simulink model "HDLOFDMMod"  (R2024a)
settings: Solver=FixedStepDiscrete  StartTime=0.0  StopTime=stopTime  RelTol=1e-3
undefined symbols (not defined in the file): CONST, dataSymbols
libraries: dspsrcs4 x2, HDL_ieee_8021513 x2, hdlsllib x1, whdlutilities x1
settings Model: DataTypeOverride=Off  Creator=cotti  LastModifiedBy=cotti
settings OptimizationCC: BlockReduction=off  ConditionallyExecuteInputs=off  DefaultParameterBehavior=Inlined  InheritOutputTypeSmallerThanSingle=on
settings DebuggingCC: ArtificialAlgebraicLoopMsg=error  SingleTaskRateTransMsg=error
settings HardwareCC: ProdBitPerPointer=32  ProdBitPerSizeT=32  ProdBitPerPtrDiffT=32  ProdLargestAtomicFloat=None  ProdIntDivRoundTo=Undefined  ProdEndianess=Unspecified  ProdWordSize=32  ProdHWDeviceType=ASIC/FPGA->ASIC/FPGA  TargetBitPerLong=64  TargetBitPerPointer=64  TargetBitPerSizeT=64  TargetBitPerPtrDiffT=64  TargetLongLongMode=on  TargetIntDivRoundTo=Zero  TargetEndianess=LittleEndian  TargetWordSize=64  TargetHWDeviceType=Custom Processor->MATLAB Host Computer  ProdEqTarget=off

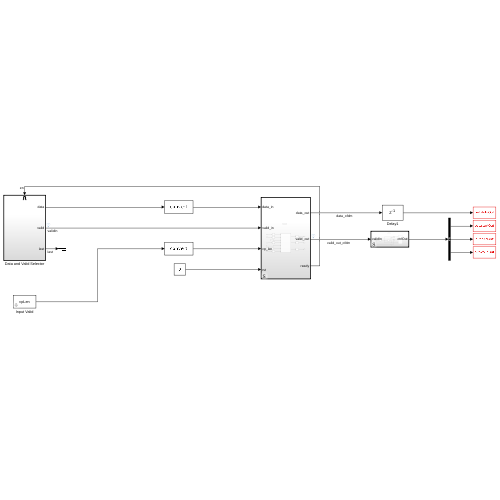
[thumbnail: Simulink's stored preview of the top-level diagram]
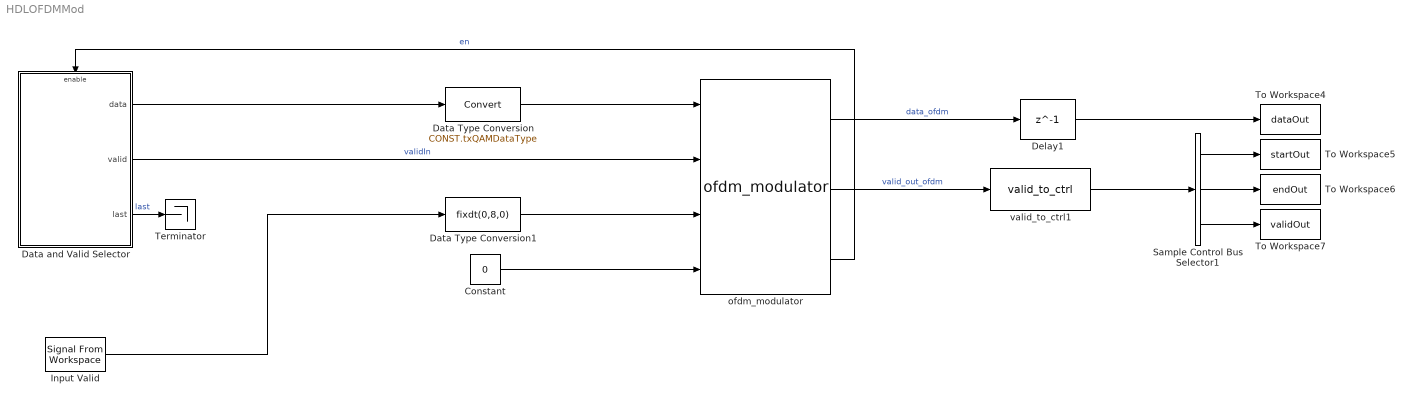
== system HDLOFDMMod ==
  Constant : Constant  Value=0  OutDataTypeStr=boolean  SampleTime=-1
  Data Type Conversion : DataTypeConversion  OutDataTypeStr=CONST.txQAMDataType  SaturateOnIntegerOverflow=off  RndMeth=Floor
  Data Type Conversion1 : DataTypeConversion  OutDataTypeStr=fixdt(0,8,0)  SaturateOnIntegerOverflow=off  RndMeth=Floor
  Data and Valid Selector : Subsystem  TreatAsAtomicUnit=on
  Delay1 : Delay  DelayLength=1  InitialCondition=0  UseCircularBuffer=on
  Input Valid : dspsrcs4/Signal From Workspace  X=cpLen  Ts=1/CONST.fPHY  nsamps=1  OutputAfterFinalValue=Holding final value  ignoreOrWarnInputAndFrameLengths=off  OutputFrames=off
  Sample Control Bus Selector1 : whdlutilities/Sample Control Bus Selector  OutputSignals=start,end,valid
  Terminator : Terminator
  To Workspace4 : ToWorkspace  VariableName=dataOut  SampleTime=1/CONST.fPHY
      settings: Save2DSignal=2-D array (concatenate along first dimension)
  To Workspace5 : ToWorkspace  VariableName=startOut  SampleTime=1/CONST.fPHY
      settings: Save2DSignal=2-D array (concatenate along first dimension)
  To Workspace6 : ToWorkspace  VariableName=endOut  SampleTime=1/CONST.fPHY
      settings: Save2DSignal=2-D array (concatenate along first dimension)
  To Workspace7 : ToWorkspace  VariableName=validOut  SampleTime=1/CONST.fPHY
      settings: Save2DSignal=2-D array (concatenate along first dimension)
  ofdm_modulator : HDL_ieee_8021513/ofdm_modulator  SystemSampleTime=-1  VariantActivationTime=update diagram  AllowFlexibleInterface=on  Latency=0  AutoFrameSizeCalculation=off
      settings: SourceProductName=HDL IEEE 8021513
  valid_to_ctrl1 : HDL_ieee_8021513/valid_to_ctrl  SystemSampleTime=-1  VariantActivationTime=update diagram  AllowFlexibleInterface=on  Latency=0  AutoFrameSizeCalculation=off
      settings: SourceProductName=HDL IEEE 8021513
  wires:
  Input Valid/1 -> Data Type Conversion1/1
  Data and Valid Selector/1(data) -> Data Type Conversion/1
  Data and Valid Selector/3(last) -> Terminator/1  "last"
  ofdm_modulator/2 -> valid_to_ctrl1/1  "valid_out_ofdm"
  valid_to_ctrl1/1 -> Sample Control Bus Selector1/1
  ofdm_modulator/1 -> Delay1/1  "data_ofdm"
  Sample Control Bus Selector1/3 -> To Workspace7/1
  Delay1/1 -> To Workspace4/1
  Sample Control Bus Selector1/1 -> To Workspace5/1
  Sample Control Bus Selector1/2 -> To Workspace6/1
  ofdm_modulator/3 -> Data and Valid Selector/Enable  "en"
  Data and Valid Selector/2(valid) -> ofdm_modulator/2  "validIn"
  Data Type Conversion/1 -> ofdm_modulator/1
  Data Type Conversion1/1 -> ofdm_modulator/3
  Constant/1 -> ofdm_modulator/4

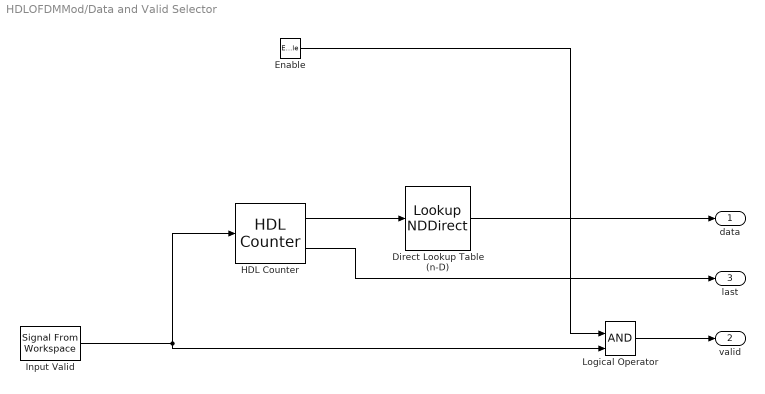
== system HDLOFDMMod/Data and Valid Selector ==
  Enable : EnablePort  ShowOutputPort=on
  Direct Lookup Table (n-D) : LookupNDDirect  NumberOfTableDimensions=1  Table=dataSymbols  DiagnosticForOutOfRangeInput=Error  TableDataTypeStr=double
  HDL Counter : hdlsllib/Sources/HDL Counter  CountType=Count limited  CountInit=0  CountStep=1  CountMax=length(dataSymbols) -1  CountFromType=Initial value  CountFrom=0  CountResetPort=off  CountLoadPort=off  CountEnbPort=on  CountDirPort=off  CountHitOutputPort=on  CountDataType=Unsigned  CountWordLen=nextpow2(length(dataSymbols))  CountFracLen=0  CountSampTime=1
  Input Valid : dspsrcs4/Signal From Workspace  X=validIn  Ts=1/CONST.fPHY  nsamps=1  OutputAfterFinalValue=Setting to zero  ignoreOrWarnInputAndFrameLengths=off  OutputFrames=off
  Logical Operator : Logic  IconShape=distinctive  AllPortsSameDT=off  OutDataTypeStr=boolean
  data : Outport  InitialOutput=0  VectorParamsAs1DForOutWhenUnconnected=off
  valid : Outport  Port=2  InitialOutput=0  VectorParamsAs1DForOutWhenUnconnected=off
  last : Outport  Port=3  VectorParamsAs1DForOutWhenUnconnected=off
  wires:
  HDL Counter/1 -> Direct Lookup Table (n-D)/1
  Input Valid/1 -> HDL Counter/1, Logical Operator/2
  Direct Lookup Table (n-D)/1 -> data/1
  HDL Counter/2 -> last/1
  Enable/1 -> Logical Operator/1
  Logical Operator/1 -> valid/1
